simulink model "VFlexP_small"  (R2026a)
settings: Solver=ode23tb  StopTime=2  FixedStep=5e-5
model workspace (MAT data in the model file):
  DCop_DCBUCK : object (value not decoded)
  Grid_CCVSC_idx = [2; 3; 4; 5; 6; 7; 8; 9; 10; 11; 12]
  Grid_CCVSCs = 1
  Grid_CCVSCs_buses = 1
  Grid_CCVSCs_toM = [0 1 0 0 0 0 0 0 0 0 0 0 ... (781 elements, 71x11)]
  Grid_C_Lines = 0
  Grid_Cbuses = [0.00666666666667 0.00666666666667]
  Grid_DC : object (value not decoded)
  Grid_DCop_DCBUCK : object (value not decoded)
  Grid_DCop_DC_PES : object (value not decoded)
  Grid_DFIGs = 1
  Grid_DFIGs_buses = 1
  Grid_DGs : string (value not decoded)
  Grid_From_buses = 1
  Grid_GFls = 1
  Grid_GFls_buses = 1
  Grid_GFr_idx = 1
  Grid_GFrs = 1
  Grid_GFrs_buses = 1
  Grid_GFrs_toM = [1; 0]
  Grid_IG_idx = 1
  Grid_IGs = 1
  Grid_IGs_buses = 1
  Grid_IGs_toM = [1; 0; 0]
  Grid_L_Lines = 0.05
  Grid_L_Loads = [0 0]
  Grid_Lines_fromM : object (value not decoded)
  Grid_Lines_toM : object (value not decoded)
  Grid_Load_buses = [1; 2]
  Grid_Load_busesDC = []
  Grid_MSGs = 1
  Grid_MSGs_buses = 1
  Grid_Nbuses = 2
  Grid_PQ_gen = 3
  Grid_Ploads = [0.0075 0.0075]
  Grid_PloadsDC = []
  Grid_Ps_lf = 0.51232912
  Grid_Qloads = [0 0]
  Grid_Qs_lf = -0.00723209333333
  Grid_R_Lines = 0.005
  Grid_R_Loads = [2 2]
  Grid_R_Loads_DC = 0
  Grid_Rcf = [150 150]
  Grid_SCs = 1
  Grid_SCs_buses = 1
  Grid_SG_idx = 1
  Grid_SGs = 1
  Grid_SGs_buses = 1
  Grid_SGs_toM = [1; 0]
  Grid_To_buses = 2
  Grid_VCVSC_idx = [1; 2; 3; 4; 5; 6; 7; 8; 9; 10; 11; 12]
  Grid_VCVSCs = 1
  Grid_VCVSCs_buses = [1; 2; 3; 6; 8; 9; 12; 58; 59; 60; 63; 65]
  Grid_VCVSCs_toM = [1 0 0 0 0 0 0 0 0 0 0 0 ... (852 elements, 71x12)]
  Grid_VSM_idx = 2
  Grid_VSMs = 1
  Grid_VSMs_buses = 1
  Grid_VSMs_toM = [0; 1]
  Grid_admitt_matrix = [2.15353135314-19.7953135314i  -1.9801980198+19.801980198i; -1.9801980198+19.801980198i  2.15353135314-19.7953135314i]
  Grid_admitt_matrix_noloads = [1.98686468647-19.7953135314i  -1.9801980198+19.801980198i; -1.9801980198+19.801980198i  1.98686468647-19.7953135314i]
  Grid_bus = [1; 2]
  Grid_busDC_complexity = 1
  Grid_busDC_complexity_PF = 2
  Grid_bus_complexity = [1 1]
  Grid_bus_complexity_PF = [1 1]
  Grid_buses_lf = 1
  Grid_conductance_matrix = 0.00666666666667
  Grid_conductance_matrix_noloads = 0.00666666666667
  Grid_fref : object (value not decoded)
  Grid_gen_static_params : mBase (value not decoded)
  Grid_iPs_lf = 1.95187031336
  Grid_iQs_lf = -138.272551792
  Grid_iadmitt_matrix = [2.88165849328-0.0982918688642i  2.87905051706-0.123273862303i; 2.87905051706-0.123273862303i  2.88165849328-0.0982918688642i]
  Grid_iadmitt_matrix_noloads = [37.5012524798-37.4874983544i  37.4987475202-37.5125016456i; 37.4987475202-37.5125016456i  37.5012524798-37.4874983544i]
  Grid_iconductance_matrix = 150
  Grid_iconductance_matrix_noloads = 150
  Grid_init_OK_bool = 1
  Grid_intconv_PF : object (value not decoded)
  Grid_lf_op : op_report (value not decoded)
  Grid_lineDC_complexity = []
  Grid_lineDC_complexity_PF = []
  Grid_line_complexity = 1
  Grid_line_complexity_PF = 3
  Grid_loadDC_complexity = []
  Grid_loadDC_complexity_PF = []
  Grid_load_complexity = [3 3]
  Grid_load_complexity_PF = [4 4]
  Grid_opDC_CCVSC : object (value not decoded)
  Grid_opDC_VSM : object (value not decoded)
  Grid_opGFr : object (value not decoded)
  Grid_opVCVSC : object (value not decoded)
  Grid_op_CCVSC : object (value not decoded)
  Grid_op_IG : object (value not decoded)
  Grid_op_SG : object (value not decoded)
  Grid_op_VSM : object (value not decoded)
  Grid_shift_lines = 0
  Grid_tap_lines = 1
  Grid_v_buses_mod = [1 1]
  LinsysParamChangeStruct : Param1 (value not decoded)
  Lline = 0.01
  Rline = 1e-05
  linsys : object (value not decoded)
values from neighbouring files (symbols this model uses):
  block_idx = evalin(mdlWks, [bvarname Generators{i} '_idx'])    [fun_init_units_callback.m]
  Fb = areas    [fun_MATPOWER_to_Excel.m]
  Fi = evalin('base', get_param(block, 'Fi'))    [fun_init_GFr.m]    (also in fun_init_intconv_DC_VSM.m)
  Lf = evalin('base', get_param(block, 'Lf'))    [fun_init_GFr.m]    (also in fun_init_intconv_DC_VSM.m)
  Rf = evalin('base', get_param(block, 'Rf'))    [fun_init_GFr.m]    (also in fun_init_intconv_DC_VSM.m)
symbols that are objects in the model workspace (value not decoded): Grid_DCop_DC_PES, Grid_DCop_DCBUCK, Grid_op_CCVSC, Grid_op_IG, Grid_op_SG, Grid_op_VSM, Grid_opDC_CCVSC, Grid_opDC_VSM, Grid_opGFr, Grid_opVCVSC
undefined symbols (not defined in the file or in its folder): block_buses_DC, CCVSC_idx, Cf, costs, costs2, DFIGs_nodes, DiscIntNeverNeededParam, entity, From_nodes, grid_linsys, Grid_op_DFIG, Grid_op_DFIG_PQ, Grid_op_MSG, Grid_op_SC, Grid_op_VCVSC, Hv, initial_states_grid, Kic, Kiv, Kp_theta, Kp_w, Kpc, Kpv, last_send, Lc, m, Matrix_flux_to_i, mD, mp, MSGs_buses, Nbuses_DC, nq, op_VCVSC, Psche, Rc, rkq1, rkq2, SCs_buses, SCs_nodes, sec_control_structure, set_asked, set_DG_up, set_extra_satur, set_sending_cost, SGs_buses, SGs_nodes, Tf, To_nodes, VI_L, VI_R, WOF_Tf, xkq1, xkq2
libraries: simulink x1045, eeGeneralControl x12, eeTransforms x1, sl_discontinuities x1
(part 5 of 50)

== system VFlexP_small/Grid/Dynamic/Generators/DFIG ==
  note: do not rename this block, conditions to initialise the generator from PF result are set on this block's output
  note: port number 1
  note: port number 2
  elec_in : Inport
  v : Inport  Port=2
  AVR_Vmeas_Filter : Subsystem  mask{T_r=1e-6}
      mask prompts: T_r "Filter time constant"
      mask Display:
      | try
      |     dpoly(1, [T_r, 1])
      | catch
      | end
  AVR_Vmeas_Filter1 : Subsystem  mask{T_r=1e-6}
      mask prompts: T_r "Filter time constant"
      mask Display:
      | try
      |     dpoly(1, [T_r, 1])
      | catch
      | end
  AVR_Vmeas_Filter2 : Subsystem  mask{T_r=1e-6}
      mask prompts: T_r "Filter time constant"
      mask Display:
      | try
      |     dpoly(1, [T_r, 1])
      | catch
      | end
  Abs : Abs  SaturateOnIntegerOverflow=off
  Assignment : Assignment  NumberOfDimensions=2  DiagnosticForDimensions=Warning  IndexOptions=Assign all,Index vector (dialog)  Indices=1,block_idx  OutputSizes=1,1
  Atan2 : Trigonometry  SCDEnableBlockLinearizationSpecification=on  Operator=atan
  Cast To Boolean : DataTypeConversion  OutDataTypeStr=boolean  SaturateOnIntegerOverflow=off  RndMeth=Floor
  Cast To Double : DataTypeConversion  OutDataTypeStr=double  SaturateOnIntegerOverflow=off  RndMeth=Floor
  Cast To Double1 : DataTypeConversion  OutDataTypeStr=double  SaturateOnIntegerOverflow=off  RndMeth=Floor
  Complex to Magnitude-Angle1 : ComplexToMagnitudeAngle  Output=Magnitude
  Constant : Constant
  Constant10 : Constant  Commented=on  Value=1.83
  Constant2 : Constant  Value=zeros(1, length(block_buses))  VectorParams1D=off
  Constant6 : Constant  Commented=on  Value=-0.2
  Constant9 : Constant  Value=-0.89
  D : Constant  Commented=on  Value=11
  Decoupling vrdqFs : Subsystem
  Display{,1..11} (12 alike) : Display
  Divide1 : Product  Inputs=*/
  Divide2 : Product  Commented=on  Inputs=*/
  Divide4 : Product  Commented=on  Inputs=*/
  For Each Subsystem : Subsystem  TreatAsAtomicUnit=on
  From54 : From  Commented=on  GotoTag=v_to_follow_own
  From55 : From  Commented=on  GotoTag=omega_r
  From61 : From  Commented=on  GotoTag=s
  GSC Control : Subsystem
  Gain1 : Gain  Gain=-1
  Gain2 : Gain  Gain=1./Lm_pu
  Gain3 : Gain  Gain=Ps_lf(block_idx)
  Gain4 : Gain  Gain=-1
  Gain5 : Gain
  Gain6 : Gain  Commented=on  Gain=2
  Gain7 : Gain  Gain=-1
  Gain9 : Gain  Gain=1./Ps_lf(block_idx)
  Goto6 : Goto  Commented=on  GotoTag=omega_r_ref
  Integrator2 : Integrator  Commented=on  InitialCondition=Grid_op_DFIG.op.States(7).x'
  Integrator3 : Integrator  InitialCondition=Grid_op_DFIG.op.States(6).x'
  Integrator4 : Integrator  InitialCondition=Grid_op_DFIG.op.States(7).x'
  Manual Switch : ManualSwitch
  Matrix Concatenate : Concatenate  NumInputs=6  Mode=Multidimensional array
  Matrix Concatenate1 : Concatenate  NumInputs=3  Mode=Multidimensional array
  Memory : Memory  InitialCondition=1
  PI Q : Subsystem
  PI TE : Subsystem
  PI v : Subsystem  Commented=on
  PLL : Subsystem
  Product{,1..17} (18 alike) : Product
  RSC Control : Subsystem
  Rblade : Constant  Commented=on  Value=28
  Real-Imag to Complex : RealImagToComplex
  Real-Imag to Complex3 : RealImagToComplex
  Reference frame transform2 : Subsystem
  Reference frame transform3 : Subsystem
  Reference frame transform4 : Subsystem
  Reference frame transform5 : Subsystem
  Rotor Mechanical : Subsystem
  Scope4 : Scope
      settings: ActiveDisplayYMinimum=0.94445  ActiveDisplayYMaximum=0.94472  DataLoggingVariableName=ScopeData2
  Selector : Selector  NumberOfDimensions=2  InputPortWidth=3  IndexOptions=Index vector (dialog),Index vector (dialog)  Indices=1,block_idx  OutputSizes=1,1
  Selector1 : Selector  NumberOfDimensions=2  InputPortWidth=9  IndexOptions=Index vector (dialog),Select all  Indices=2,1  OutputSizes=1,1
  Selector2 : Selector  NumberOfDimensions=2  InputPortWidth=9  IndexOptions=Index vector (dialog),Select all  Indices=1,1  OutputSizes=1,1
  Selector3 : Selector  NumberOfDimensions=2  InputPortWidth=3  IndexOptions=Index vector (dialog),Index vector (dialog)  Indices=2,block_idx  OutputSizes=1,1
  Selector4 : Selector  NumberOfDimensions=2  InputPortWidth=3  IndexOptions=Index vector (dialog),Index vector (dialog)  Indices=3,block_idx  OutputSizes=1,1
  Selector5 : Selector  NumberOfDimensions=2  InputPortWidth=3  IndexOptions=Index vector (dialog),Index vector (dialog)  Indices=4,block_idx  OutputSizes=1,1
  Selector6 : Selector  NumberOfDimensions=2  InputPortWidth=3  IndexOptions=Index vector (dialog),Index vector (dialog)  Indices=5,block_idx  OutputSizes=1,1
  Selector7 : Selector  NumberOfDimensions=2  InputPortWidth=3  IndexOptions=Index vector (dialog),Index vector (dialog)  Indices=1,block_buses  OutputSizes=1,1
  Selector8 : Selector  NumberOfDimensions=2  InputPortWidth=3  IndexOptions=Index vector (dialog),Index vector (dialog)  Indices=2,block_buses  OutputSizes=1,1
  Signal Specification : SignalSpecification  Dimensions=[6 length(buses_lf)]
  Signal Specification1 : SignalSpecification  Dimensions=[3 length(block_buses)]
  Slip : Subsystem  Commented=on
      settings: PortSchema="{\"entries\":[{\"content\":{\"sides\":[{\"content\":{\"connectorIds\":[\"In1\",\"In2\"]},\"type\":\"ConnectorPlacement.EquallySpacedRectSide\",\"uuid\":\"76dc537b-974c-49aa-a996-6680dce67c21\"},{\"content\":{\"connectorIds\":[\"Out1\",\"Out2\"],\"side\":\"RIGHT\"},\"type\":\"ConnectorPlacement.EquallySpacedRectSide\",\"uuid\":\"b6b8ef66-c2c7-4653-a511-fa1c360be79f\"},{\"content\":{\"connectorIds\":[],\"side\":\"TOP\"},\"type\":\"ConnectorPlacement.EquallySpacedRectSide\",\"uuid\":\"e58a1e6b-6a60-4748-900e-908d64e83c02\"},{\"content\":{\"connectorIds\":[\"In3\"],\"side\":\"BOTTOM\"},\"type\":\"ConnectorPlacement.EquallySpacedRectSide\",\"uuid\":\"479d910e-b2a0-4bf0-91fd-3472aae41677\"}]},\"type\":\"ConnectorPlacement.EquallySpacedConnector\",\"uuid\":\"d6647aa7-5f1b-4486-ad87-47217a09b45e\"}],\"packageUris\":[\"http://schema.mathworks.com/mf0/Connector/R2020b\"],\"version\":\"1.0\"}"
  Stator circuit : Subsystem
  Subsystem : Subsystem
  Subsystem1 : Subsystem
  Sum : Sum  Inputs=-|-|-
  Sum{1,5..6,10..11,13} (6 alike) : Sum  Inputs=|-+
  Sum{4,9,12,14} (4 alike) : Sum  Inputs=|++
  Sum2 : Sum  Inputs=-|-|-
  Sum3 : Sum  Commented=on  Inputs=|+-
  Sum7 : Sum  Inputs=|+-
  TF_DELAY : Subsystem  Commented=on  mask{T_s=0.0001}
      mask prompts: T_s "Filter time constant"
      mask Display:
      | try
      |     dpoly(1, [T_s, 1])
      | catch
      | end
  TF_DELAY1 : Subsystem  mask{T_s=20E-3}
      mask prompts: T_s "Filter time constant"
      mask Display:
      | try
      |     dpoly(1, [T_s, 1])
      | catch
      | end
  Terminator{,1,3..8} (8 alike) : Terminator
  Vc control : Subsystem
  Vwind1 : Constant  Commented=on  Value=6
  Zero1 : Constant  Value=zeros(6, length(buses_lf))  VectorParams1D=off  OutDataTypeStr=Inherit: Inherit via back propagation
  connect : Subsystem
  lambda_opt : Gain  Commented=on  Gain=8
  psi->i1 : Subsystem
  tm : Integrator  InitialCondition=Grid_op_DFIG.op.States(24).x'  LimitOutput=on  UpperSaturationLimit=0  LowerSaturationLimit=-1
  trim_output : Subsystem
  w_ref_TF : Subsystem  Commented=on  mask{T_s=0.05}
      mask prompts: T_s "Filter time constant"
      mask Display:
      | try
      |     dpoly(1, [T_s, 1])
      | catch
      | end
  elec_out : Outport
  i : Outport  Port=2
  wires:
  From61/1 -> Slip/2(s)
  TF_DELAY/1(out) -> Gain6/1
  From55/1 -> TF_DELAY/1(in)
  D/1 -> Divide4/2
  Subsystem1/1(te) -> [te], Display10/1
  Divide4/1 -> w_ref_TF/1(in)
  w_ref_TF/1(out) -> Goto6/1
  Rblade/1 -> Divide2/2
  lambda_opt/1 -> Divide2/1
  Vwind1/1 -> Divide4/1, lambda_opt/1
  Sum7/1 -> PI Q/1(in)
  Sum4/1 -> AVR_Vmeas_Filter1/1(in)  "v"
  Sum5/1 -> AVR_Vmeas_Filter2/1(in)  "v"
  Real-Imag to Complex3/1 -> Complex to Magnitude-Angle1/1
  [v_q_PCC] -> Real-Imag to Complex3/2
  Complex to Magnitude-Angle1/1 -> AVR_Vmeas_Filter/1(in)  "v"
  [v_d_PCC] -> Real-Imag to Complex3/1
  Product5/1 -> Sum5/1
  [v_d_PCC] -> Product1/1, Product5/1  "vod"
  Product3/1 -> Sum4/2
  [id_out] -> Product1/2, Product6/2  "iod"
  [v_q_PCC] -> Product6/1, Product3/1  "voq"
  Product6/1 -> Sum5/2
  Product1/1 -> Sum4/1
  [iq_out] -> Product3/2, Product5/2  "ioq"
  tm/1 -> Manual Switch/1
  Signal Specification/1 -> elec_out/1
  Gain4/1 -> Reference frame transform3/2(theta)
  [vaq] -> Stator circuit/6(vaq)
  Constant9/1 -> Manual Switch/2
  Sum/1 -> Reference frame transform5/1(in_d)
  Sum2/1 -> Reference frame transform5/3(in_q)
  PLL/1(theta_rad_pll) -> [theta], Terminator1/1
  For Each Subsystem/1(Out1) -> i/1
  Reference frame transform5/1(out_d) -> connect/1(id), [id_out]
  Product/1 -> Sum1/1
  [v_d_PCC] -> Stator circuit/1(vsd)
  trim_output/2(Out2) -> Terminator6/1
  ? -> Sum2/3
  [vrd_] -> Decoupling vrdqFs/2(Vrd')
  [vad] -> Stator circuit/5(vad)
  Selector5/1 -> [Q_s_to_follow_own]
  [iad] -> GSC Control/4(iad)
  Vc control/1(iad_ref) -> [iad_ref]
  psi->i1/5(irq) -> [irq], Subsystem1/3(irq)
  Real-Imag to Complex/1 -> Abs/1
  [vrd] -> Vc control/2(vrd)
  [vad] -> Vc control/6(vad)
  [te] -> Rotor Mechanical/1(te)
  [omega_ref] -> Terminator/1  "ref_omega"
  [vrd] -> Stator circuit/3(vrd)
  Assignment/1 -> Signal Specification/1
  Reference frame transform2/2(vrq) -> [vrq]
  [v_q_PCC] -> PLL/1(vdq0_meas)
  Decoupling vrdqFs/1(vrd_Fs) -> Reference frame transform2/1(vrd_Fs)
  GSC Control/1(vad) -> [vad]
  [v_q_PCC] -> Stator circuit/2(vsq)
  psi->i1/6(iad) -> [iad]
  [iaq] -> Vc control/9(iaq)
  Selector2/1 -> Divide1/2, Real-Imag to Complex/1
  GSC Control/2(vaq) -> [vaq]
  [vsq] -> GSC Control/2(vsq)
  RSC Control/2(vrq') -> [vrq_]
  RSC Control/1(vrd') -> [vrd_]
  [phi] -> Gain1/1
  [vrq] -> Vc control/3(vrq)
  Divide1/1 -> Atan2/1
  [ws] -> Decoupling vrdqFs/4(ws)
  Reference frame transform2/1(vrd) -> [vrd]
  PLL/2(omega_pu_pll) -> Terminator3/1
  [vrq_] -> Decoupling vrdqFs/6(vrq')
  psi->i1/3(isq) -> [isq]
  [iad_ref] -> GSC Control/3(iad_ref)
  ? -> Sum/3
  PLL/3(Freq_Hz_pll) -> Terminator4/1
  Constant/1 -> Vc control/1(Vc_2_ref)
  [iad] -> Vc control/8(iad)
  Gain2/1 -> Decoupling vrdqFs/5(ism)
  [vdout] -> Reference frame transform3/1(in_d)
  [theta] -> Gain4/1
  Gain9/1 -> Matrix Concatenate/2
  Reference frame transform3/2(out_q) -> [vsq], [v_q_PCC]
  [P_s] -> Gain9/1  "P_s"
  [isd] -> Sum/1
  psi->i1/4(ird) -> [ird], Subsystem1/2(ird)
  Matrix Concatenate1/1 -> Signal Specification1/1
  trim_output/4(Out4) -> Terminator8/1
  Selector8/1 -> [vqout], trim_output/4(vq)
  Constant2/1 -> Matrix Concatenate1/3
  [irq] -> Reference frame transform4/3(irq)
  [vqout] -> Reference frame transform3/3(in_q)
  trim_output/3(Out3) -> Terminator7/1
  Cast To Boolean/1 -> [connect]
  [ws] -> Stator circuit/8(ws)
  v/1 -> Selector8/1, Selector7/1
  Rotor Mechanical/1(s) -> Product/1, [s]
  [i] -> Stator circuit/7(i)
  Signal Specification1/1 -> For Each Subsystem/1(In1)
  [vsd] -> GSC Control/1(vsd)
  Reference frame transform4/2(out_q) -> RSC Control/4(irq_Fs_meas), Decoupling vrdqFs/1(irq_Fs)
  Atan2/1 -> [phi], Display2/1
  [ws] -> GSC Control/7(ws)
  Selector7/1 -> trim_output/3(vd), [vdout]
  Gain5/1 -> Reference frame transform5/2(theta)
  elec_in/1 -> Selector6/1, Selector5/1, Selector4/1, Selector3/1, Selector/1
  connect/2(iq_real) -> trim_output/2(iq), Matrix Concatenate1/2
  [connect] -> Cast To Double1/1
  Cast To Double/1 -> Matrix Concatenate/6
  Cast To Double1/1 -> Matrix Concatenate/5
  [phi] -> Reference frame transform2/2(phi)
  Selector6/1 -> Cast To Boolean/1
  [Q_s] -> Matrix Concatenate/4  "Q_s"
  connect/1(id_real) -> trim_output/1(id), Matrix Concatenate1/1
  [ird] -> Reference frame transform4/1(ird)
  psi->i1/7(iaq) -> [iaq]
  [vrq] -> Stator circuit/4(vrq)
  psi->i1/1(i) -> Display1/1, [i]
  trim_output/1(Out1) -> Terminator5/1
  [ws] -> Matrix Concatenate/1  "omega"
  Zero1/1 -> Assignment/1
  Selector/1 -> [omega_to_follow_own]
  Selector3/1 -> Gain3/1
  Selector4/1 -> [v_to_follow_own]
  Gain3/1 -> [P_s_to_follow_own]
  [vaq] -> Vc control/7(vaq)
  [ird] -> Vc control/4(ird)
  Matrix Concatenate/1 -> Assignment/2
  [iaq] -> GSC Control/6(iaq)
  [isq] -> Sum2/1
  [omega_ref] -> Rotor Mechanical/3(ws), Product/2, [ws], Sum1/2
  Reference frame transform5/2(out_q) -> connect/2(iq), [iq_out]
  [theta] -> Gain5/1
  psi->i1/2(isd) -> [isd]
  Stator circuit/1(psi) -> Display/1, psi->i1/1(psi), Subsystem1/1(psisdq), Selector1/1, Selector2/1
  [connect] -> connect/3(connect)
  [s] -> Stator circuit/9(s)
  Decoupling vrdqFs/2(vrq_Fs) -> Reference frame transform2/3(vrq_Fs)
  Reference frame transform3/1(out_d) -> [vsd], [v_d_PCC]
  [s] -> Decoupling vrdqFs/3(s)
  [iad] -> Sum/2
  AVR_Vmeas_Filter/1(out) -> [Vt_mod], Matrix Concatenate/3  "v"
  Selector1/1 -> Divide1/1, Real-Imag to Complex/2
  [connected] -> Memory/1
  [irq] -> Vc control/5(irq)
  connect/3(connected) -> [connected]
  [iaq] -> Sum2/2
  Gain1/1 -> Reference frame transform4/2(phi)
  Memory/1 -> Cast To Double/1
  [isd] -> Product4/2, Product9/2  "iod"
  [isq] -> Product7/2, Product8/2  "ioq"
  Product9/1 -> Sum10/2
  Product7/1 -> Sum9/2
  [v_d_PCC] -> Product4/1, Product8/1  "vod"
  Sum10/1 -> [Q_stator], Display7/1  "v"
  [v_q_PCC] -> Product9/1, Product7/1  "voq"
  Product4/1 -> Sum9/1
  Sum9/1 -> Display8/1, [P_stator]  "v"
  Product8/1 -> Sum10/1
  Product12/1 -> Sum11/1
  Sum12/1 -> [P_rotor], Display6/1  "v"
  Product10/1 -> Sum12/1
  [vrq] -> Product11/1, Product13/1  "voq"
  Sum11/1 -> Display5/1, [Q_rotor]  "v"
  [vrd] -> Product12/1, Product10/1  "vod"
  Product11/1 -> Sum12/2
  Product13/1 -> Sum11/2
  [irq] -> Product12/2, Product11/2  "ioq"
  [ird] -> Product13/2, Product10/2  "iod"
  [iad] -> Product14/2, Product17/2  "iod"
  [iaq] -> Product15/2, Product16/2  "ioq"
  Product17/1 -> Sum13/2
  Product15/1 -> Sum14/2
  [vad] -> Product14/1, Product16/1  "vod"
  Sum13/1 -> [Q_gsc], Display3/1  "v"
  [vaq] -> Product17/1, Product15/1  "voq"
  Product14/1 -> Sum14/1
  Sum14/1 -> Display4/1, [P_gsc]  "v"
  Product16/1 -> Sum13/1
  Constant6/1 -> Slip/1(s_ref)
  Slip/2(Te) -> ?
  Integrator3/1 -> Sum7/2
  AVR_Vmeas_Filter1/1(out) -> [P_s], Display9/1  "v"
  AVR_Vmeas_Filter2/1(out) -> [Q_s]  "v"
  Subsystem/1(Out1) -> Gain7/1
  Product2/1 -> Subsystem/1(omega_r)
  [omega_r] -> TF_DELAY1/1(in)
  Sum3/1 -> PI v/1(in)
  From54/1 -> Sum3/1
  Sum1/1 -> [omega_r], Scope4/1
  Abs/1 -> Gain2/1
  Integrator2/1 -> Sum3/2
  Gain7/1 -> Display11/1, [Te_ref]
  [Te_ref] -> Sum6/1
  [te] -> Sum6/2
  Sum6/1 -> PI TE/1(in)
  TF_DELAY1/1(out) -> Product2/2, Product2/1
  [Q_s_to_follow_own] -> Sum7/1
  Integrator4/1 -> GSC Control/5(iaq_ref)
  PI TE/1(out) -> RSC Control/3(irq_Fs_ref)
  Reference frame transform4/1(out_d) -> RSC Control/2(ird_Fs_meas), Decoupling vrdqFs/7(ird_Fs)
  PI Q/1(out) -> RSC Control/1(ird_Fs_ref)
  Manual Switch/1 -> Rotor Mechanical/2(tm)

== system VFlexP_small/Grid/Dynamic/Generators/GFl ==
  note: do not rename this block, conditions to initialise the generator from PF result are set on this block's output
  note: port number 1
  note: port number 2
  elec_in : Inport
  v : Inport  Port=2
  Assignment : Assignment  NumberOfDimensions=2  DiagnosticForDimensions=Warning  IndexOptions=Assign all,Index vector (dialog)  Indices=1,block_idx  OutputSizes=1,1
  CC : Subsystem  Variant=on  VariantControlMode=label  LabelModeActiveChoice=static
  Cast To Boolean1 : DataTypeConversion  OutDataTypeStr=boolean  SaturateOnIntegerOverflow=off  RndMeth=Floor
  Cast To Double : DataTypeConversion  OutDataTypeStr=double  SaturateOnIntegerOverflow=off  RndMeth=Floor
  Cast To Double1 : DataTypeConversion  OutDataTypeStr=double  SaturateOnIntegerOverflow=off  RndMeth=Floor
  Cast To Double2 : DataTypeConversion  OutDataTypeStr=double  SaturateOnIntegerOverflow=off  RndMeth=Floor
  Complex to Magnitude-Angle : ComplexToMagnitudeAngle  Output=Angle
  Complex to Magnitude-Angle1 : ComplexToMagnitudeAngle  Output=Magnitude
  Constant : Constant  Value=zeros(1, length(block_buses))  VectorParams1D=off
  For Each Subsystem : Subsystem  TreatAsAtomicUnit=on
  Gain : Gain  Gain=-1
  Gain3 : Gain  Commented=through  Gain=iQs_lf(CCVSC_idx)
  Gain4 : Gain  Commented=through  Gain=iPs_lf(CCVSC_idx)
  LPF : Subsystem
  LPF1 : Subsystem
  LPF2 : Subsystem
  LPF3 : Subsystem
  LPF_d : Subsystem  Commented=through
  LPF_q : Subsystem  Commented=through
  Matrix Concatenate : Concatenate  NumInputs=6  Mode=Multidimensional array
  Matrix Concatenate1 : Concatenate  NumInputs=3  Mode=Multidimensional array
  Memory : Memory  InitialCondition=1
  Memory1 : Memory  InitialCondition=1
  Memory2 : Memory  InitialCondition=1
  PC : Subsystem
      settings: PortSchema="{\"entries\":[{\"content\":{\"sides\":[{\"content\":{\"connectorIds\":[\"In1\",\"In2\",\"In3\",\"In4\"]},\"type\":\"ConnectorPlacement.EquallySpacedRectSide\",\"uuid\":\"7748ce6f-2dcc-431c-b3ea-0be9c3088b1d\"},{\"content\":{\"connectorIds\":[\"In5\",\"Out1\",\"Out2\"],\"side\":\"RIGHT\"},\"type\":\"ConnectorPlacement.EquallySpacedRectSide\",\"uuid\":\"af86fd8d-043b-4d20-8ee8-e7a977d706a8\"},{\"content\":{\"connectorIds\":[],\"side\":\"TOP\"},\"type\":\"ConnectorPlacement.EquallySpacedRectSide\",\"uuid\":\"807e0dc6-0d59-4ea5-9557-3ccfd29c2ad0\"}]},\"type\":\"ConnectorPlacement.EquallySpacedConnector\",\"uuid\":\"c7fe00c5-0a0a-4038-b7ac-e659fb2aa4a7\"}],\"packageUris\":[\"http://schema.mathworks.com/mf0/Connector/R2020b\"],\"version\":\"1.0\"}"
  PLL : Subsystem  Variant=on  VariantControlMode=label  LabelModeActiveChoice=dynamic
  Product{,1..3} (4 alike) : Product
  Real-Imag to Complex : RealImagToComplex
  Real-Imag to Complex1 : RealImagToComplex
  Reference frame transform3 : Subsystem
  Reference_frame_transform1 : Subsystem
  Selector : Selector  NumberOfDimensions=2  InputPortWidth=3  IndexOptions=Index vector (dialog),Index vector (dialog)  Indices=1,block_idx  OutputSizes=1,1
  Selector1 : Selector  NumberOfDimensions=2  InputPortWidth=3  IndexOptions=Index vector (dialog),Index vector (dialog)  Indices=2,block_idx  OutputSizes=1,1
  Selector2 : Selector  NumberOfDimensions=2  InputPortWidth=3  IndexOptions=Index vector (dialog),Index vector (dialog)  Indices=3,block_idx  OutputSizes=1,1
  Selector3 : Selector  NumberOfDimensions=2  InputPortWidth=3  IndexOptions=Index vector (dialog),Index vector (dialog)  Indices=4,block_idx  OutputSizes=1,1
  Selector4 : Selector  NumberOfDimensions=2  InputPortWidth=3  IndexOptions=Index vector (dialog),Index vector (dialog)  Indices=5,block_idx  OutputSizes=1,1
  Selector5 : Selector  NumberOfDimensions=2  InputPortWidth=3  IndexOptions=Index vector (dialog),Index vector (dialog)  Indices=1,block_buses  OutputSizes=1,1
  Selector6 : Selector  NumberOfDimensions=2  InputPortWidth=3  IndexOptions=Index vector (dialog),Index vector (dialog)  Indices=2,block_buses  OutputSizes=1,1
  Selector7 : Selector  InputPortWidth=length(fref.ref_units)  IndexOptions=Index vector (dialog)  Indices=block_fref  OutputSizes=1
  Signal Specification : SignalSpecification  Dimensions=[6 length(buses_lf)]
  Signal Specification1 : SignalSpecification  Dimensions=[3 length(block_buses)]
  Sum : Sum  Inputs=|++
  Sum1 : Sum  Inputs=|-+
  Terminator{,3..5} (4 alike) : Terminator
  Zero1 : Constant  Value=zeros(6, length(buses_lf))  VectorParams1D=off  OutDataTypeStr=Inherit: Inherit via back propagation
  connect : Subsystem
  trim_output : Subsystem
  elec_out : Outport
  i : Outport  Port=2
  wires:
  LPF_q/1(Out1) -> Gain3/1
  LPF_d/1(Out1) -> Gain4/1
  [voutangle] -> PLL/1(voutangle)
  [Q_s_to_follow_own] -> PC/4(vodi2)
  [P_s_to_follow_own] -> PC/3(vodi1)
  connect/3(connected) -> Cast To Double/1
  CC/2(iqiref) -> Reference_frame_transform1/2(qin)  "ioq"
  CC/1(idiref) -> Reference_frame_transform1/1(din)  "iod"
  Reference frame transform3/2(out_q) -> [voq]
  PLL/1(theta) -> [theta]
  [omega_ref] -> Selector7/1
  [voq] -> PLL/2(vq)
  [theta] -> Reference_frame_transform1/3(theta)
  Gain/1 -> Reference frame transform3/2(theta)
  [theta] -> Gain/1
  PC/2(Output1) -> CC/2(iqref)  "ioq"
  PC/1(Output) -> CC/1(idref)  "iod"
  [v_q_PCC] -> Product3/1  "voq"
  [v_d_PCC] -> Product2/1  "vod"
  [ioq] -> Product1/2  "ioq"
  [iod] -> Product/2  "iod"
  [v_d_PCC] -> Product/1  "vod"
  Gain3/1 -> [Q_s]
  Gain4/1 -> [P_s]
  Product/1 -> Sum/1
  Product3/1 -> Sum1/2
  Product1/1 -> Sum/2
  Product2/1 -> Sum1/1
  [ioq] -> Product2/2  "ioq"
  [iod] -> Product3/2  "iod"
  Sum1/1 -> LPF_q/1(In1)
  Sum/1 -> LPF_d/1(In1)
  [v_q_PCC] -> Product1/1  "voq"
  Reference frame transform3/1(out_d) -> [vod]  "v CCVSC"
  [voq] -> PC/2(voq), CC/4(voq)
  [vod] -> PC/1(vodi), CC/3(vod)
  Real-Imag to Complex/1 -> Complex to Magnitude-Angle/1
  Complex to Magnitude-Angle/1 -> [voutangle]
  PLL/2(omega_point) -> PC/5(omega), CC/5(omega), [omega]  "\\omega CCVSC"
  Reference_frame_transform1/2(qout) -> connect/2(iq)
  Reference_frame_transform1/1(dout) -> connect/1(id)
  [vqout] -> LPF3/1(In1)
  Selector3/1 -> [Q_s_to_follow_own]
  Selector2/1 -> [v_to_follow_own]
  Selector/1 -> [omega_to_follow_own]
  [omega] -> Matrix Concatenate/1  "omega"
  [P_s] -> Matrix Concatenate/2  "P_s"
  [Q_s] -> Matrix Concatenate/4  "Q_s"
  [connected] -> Memory/1
  [connect] -> Memory1/1
  Cast To Double/1 -> [connected]
  [connect] -> connect/3(connect)
  [vdout] -> LPF2/1(In1)
  connect/1(id_real) -> [iod], trim_output/1(id), Matrix Concatenate1/1
  connect/2(iq_real) -> [ioq], trim_output/2(iq), Matrix Concatenate1/2
  LPF3/1(Out1) -> [v_q_PCC]
  LPF2/1(Out1) -> [v_d_PCC]
  [v_d_PCC] -> Real-Imag to Complex1/1  "vod"
  [v_q_PCC] -> Real-Imag to Complex1/2  "voq"
  Real-Imag to Complex1/1 -> Complex to Magnitude-Angle1/1
  Complex to Magnitude-Angle1/1 -> Matrix Concatenate/3
  [v_d_PCC] -> LPF/1(In1)  "vod"
  [v_q_PCC] -> LPF1/1(In1)  "voq"
  Selector4/1 -> Cast To Boolean1/1
  Cast To Boolean1/1 -> Memory2/1
  Cast To Double1/1 -> Matrix Concatenate/5
  Cast To Double2/1 -> Matrix Concatenate/6
  Zero1/1 -> Assignment/1
  Signal Specification/1 -> elec_out/1
  Assignment/1 -> Signal Specification/1
  Matrix Concatenate/1 -> Assignment/2
  elec_in/1 -> Selector4/1, Selector3/1, Selector2/1, Selector1/1, Selector/1
  Matrix Concatenate1/1 -> Signal Specification1/1
  Signal Specification1/1 -> For Each Subsystem/1(In1)
  Constant/1 -> Matrix Concatenate1/3
  For Each Subsystem/1(Out1) -> i/1
  trim_output/1(Out1) -> Terminator/1
  trim_output/3(Out3) -> Terminator4/1
  trim_output/2(Out2) -> Terminator3/1
  trim_output/4(Out4) -> Terminator5/1
  Selector5/1 -> trim_output/3(vd), [vdout]
  Selector6/1 -> trim_output/4(vq), [vqout]
  v/1 -> Selector6/1, Selector5/1
  Memory/1 -> Cast To Double2/1
  Selector1/1 -> [P_s_to_follow_own]
  Memory1/1 -> Cast To Double1/1
  Memory2/1 -> [connect]
  LPF/1(Out1) -> Reference frame transform3/1(in_d), Real-Imag to Complex/1
  LPF1/1(Out1) -> Real-Imag to Complex/2, Reference frame transform3/3(in_q)
  Selector7/1 -> PLL/3(omega)

== system VFlexP_small/Grid/Dynamic/Generators/GFr ==
  note: port number 1
  note: do not rename this block, conditions to initialise the generator from PF result are set on this block's output
  note: port number 2
  elec_in : Inport
  v : Inport  Port=2
  AND : Logic  IconShape=distinctive  AllPortsSameDT=off  OutDataTypeStr=boolean
  AND1 : Logic  IconShape=distinctive  AllPortsSameDT=off  OutDataTypeStr=boolean
  AND2 : Logic  IconShape=distinctive  AllPortsSameDT=off  OutDataTypeStr=boolean
  Abs{,1..3} (4 alike) : Abs  ZeroCross=off  SaturateOnIntegerOverflow=off
  Assignment : Assignment  NumberOfDimensions=2  DiagnosticForDimensions=Warning  IndexOptions=Assign all,Index vector (dialog)  Indices=1,block_idx  OutputSizes=1,1
  Atan2 : Trigonometry  Operator=atan2
  Cast To Boolean : DataTypeConversion  OutDataTypeStr=boolean  SaturateOnIntegerOverflow=off  RndMeth=Floor
  Cast To Double : DataTypeConversion  OutDataTypeStr=double  SaturateOnIntegerOverflow=off  RndMeth=Floor
  Cast To Double1 : DataTypeConversion  OutDataTypeStr=double  SaturateOnIntegerOverflow=off  RndMeth=Floor
  Cast To Double2 : DataTypeConversion  OutDataTypeStr=double  SaturateOnIntegerOverflow=off  RndMeth=Floor
  Compare To Constant : simulink/Logic and Bit Operations/Compare To Constant  relop=<=  const=0.001  OutDataTypeStr=boolean  ZeroCross=off
  Compare To Constant1 : simulink/Logic and Bit Operations/Compare To Constant  relop=<=  const=0.01  OutDataTypeStr=boolean  ZeroCross=off
  Compare To Constant2 : simulink/Logic and Bit Operations/Compare To Constant  relop=<=  const=0.2  OutDataTypeStr=boolean  ZeroCross=off
  Compare To Constant3 : simulink/Logic and Bit Operations/Compare To Constant  relop=>  const=4  OutDataTypeStr=boolean  ZeroCross=off
  Complex to Magnitude-Angle1 : ComplexToMagnitudeAngle  Output=Magnitude
  Complex to Real-Imag : ComplexToRealImag
  Conjugate : Math  Operator=conj  SignedPower=on  RndMeth=Zero
  Constant : Constant  Value=zeros(1, length(block_buses))  VectorParams1D=off
  Constant1 : Constant  Value=Grid_opVCVSC.Pd
  For Each Subsystem : Subsystem  TreatAsAtomicUnit=on
  Gain : Gain  Gain=mD
  Gain1 : Gain  Gain=-1
  Gain2 : Gain  Gain=-1
  Integrator : Integrator  ExternalReset=falling  InitialCondition=Grid_opGFr.IntConnect
  LPF : Subsystem  Commented=through
  LPF1 : Subsystem  Commented=through
  LPF_P : Subsystem
  LPF_omega : Subsystem
  LPF_v : Subsystem
  Matrix Concatenate : Concatenate  NumInputs=6  Mode=Multidimensional array
  Matrix Concatenate1 : Concatenate  NumInputs=3  Mode=Multidimensional array
  Memory : Memory  InitialCondition=1
  Memory1 : Memory  InitialCondition=1
  Memory2 : Memory  InitialCondition=1
  NOT1 : Logic  Operator=NOT  IconShape=distinctive  AllPortsSameDT=off  OutDataTypeStr=boolean
  OR : Logic  Operator=OR  Inputs=3  IconShape=distinctive  AllPortsSameDT=off  OutDataTypeStr=boolean
  PC : Subsystem  mask(PC_VCVSC){Tf=Tf, mp=mp, nq=nq}
      mask prompts: Tf "Low-pass filter time constant (s)"; mp "Droop coefficient mp"; nq "Droop coefficient nq"
      mask help: Power controller of a grid-forming converter, including the droop control and low-pass filters for the power measurements.
      mask init: same as VFlexP_small/Grid/Dynamic/DCAC converters/DC_VCVSC/PC
  PI_synchro_f : Subsystem
  PI_synchro_v : Subsystem
  Product : Product
  Product1 : Product  OutDataTypeStr=double
  Product2 : Product  OutDataTypeStr=double
  Product3 : Product
  RL out : Subsystem  Variant=on  VariantControlMode=label  LabelModeActiveChoice=dynamic  mask{dynamic=Dynamic, R=R_out, L=L_out}
      mask prompts: dynamic "Dynamic behavior"; R "Series resistance (p.u.)"; L "Inductance (p.u.)"
      mask init:
      | invL = 1./L;
      | vssBlk = gcb;
      | switch dynamic
      |     case "Static"
      |         set_param(vssBlk, 'LabelModeActiveChoice', 'static');
      |     case "Dynamic"
      |         set_param(vssBlk, 'LabelModeActiveChoice', 'dynamic');
      |     case "Static omega"
      |         set_param(vssBlk, 'LabelModeActiveChoice', 'static_omega');
      | end
      mask TypeOptions dynamic: Static | Dynamic | Static omega
  Real-Imag to Complex : RealImagToComplex
  Real-Imag to Complex1 : RealImagToComplex
  Real-Imag to Complex3 : RealImagToComplex
  Reference frame transform1 : Subsystem
  Reference frame transform2 : Subsystem
  Reference frame transform3 : Subsystem
  Scope : Scope
      settings: ActiveDisplayYMinimum=0.9  ActiveDisplayYMaximum=1.1
  Selector : Selector  NumberOfDimensions=2  InputPortWidth=3  IndexOptions=Index vector (dialog),Index vector (dialog)  Indices=1,block_idx  OutputSizes=1,1
  Selector1 : Selector  NumberOfDimensions=2  InputPortWidth=3  IndexOptions=Index vector (dialog),Index vector (dialog)  Indices=2,block_idx  OutputSizes=1,1
  Selector2 : Selector  NumberOfDimensions=2  InputPortWidth=3  IndexOptions=Index vector (dialog),Index vector (dialog)  Indices=3,block_idx  OutputSizes=1,1
  Selector3 : Selector  NumberOfDimensions=2  InputPortWidth=3  IndexOptions=Index vector (dialog),Index vector (dialog)  Indices=4,block_idx  OutputSizes=1,1
  Selector4 : Selector  NumberOfDimensions=2  InputPortWidth=3  IndexOptions=Index vector (dialog),Index vector (dialog)  Indices=5,block_idx  OutputSizes=1,1
  Selector5 : Selector  NumberOfDimensions=2  InputPortWidth=3  IndexOptions=Index vector (dialog),Index vector (dialog)  Indices=1,block_buses  OutputSizes=1,1
  Selector6 : Selector  NumberOfDimensions=2  InputPortWidth=3  IndexOptions=Index vector (dialog),Index vector (dialog)  Indices=2,block_buses  OutputSizes=1,1
  Selector7 : Selector  InputPortWidth=length(fref.ref_units)  IndexOptions=Index vector (dialog)  Indices=block_fref  OutputSizes=1
  Selector8 : Selector  InputPortWidth=length(fref.ref_units)  IndexOptions=Index vector (dialog)  Indices=block_fref  OutputSizes=1
  Signal Specification : SignalSpecification  Dimensions=[6 length(buses_lf)]
  Signal Specification1 : SignalSpecification  Dimensions=[3 length(block_buses)]
  Sum : Sum  Inputs=|+-
  Sum1 : Sum  Inputs=|++
  Sum11 : Sum  Inputs=|++
  Sum12 : Sum  Inputs=|++
  Sum2 : Sum  Inputs=-+|
  Sum3 : Sum  Inputs=|+-
  Sum4 : Sum  Inputs=|+-
  Sum8 : Sum  Inputs=++|
  Switch2 : Switch  Criteria=u2 > Threshold  SaturateOnIntegerOverflow=off  InputSameDT=off
  Switch3 : Switch  Criteria=u2 > Threshold  SaturateOnIntegerOverflow=off  InputSameDT=off
  Terminator{,1..5} (6 alike) : Terminator
  VCC : Subsystem  Variant=on  VariantControlMode=label  LabelModeActiveChoice=static
  VI : Subsystem  mask{L=VI_L, R=VI_R, Tf=WOF_Tf}
      mask prompts: L "Inductance (pu)"; R "Resistance (pu)"; Tf "WOF time constant (s)"
      mask init: same as VFlexP_small/Grid/Dynamic/DCAC converters/DC_VCVSC/VI
  Zero : Constant  Value=0  OutDataTypeStr=Inherit: Inherit via back propagation
  Zero1 : Constant  Value=zeros(6, length(buses_lf))  VectorParams1D=off  OutDataTypeStr=Inherit: Inherit via back propagation
  connect : Subsystem
  frame : Integrator  InitialCondition=Grid_opGFr.frame  IgnoreLimit=on
  iV : Integrator  InitialCondition=Grid_opGFr.iV
  trim_output : Subsystem
  vod : Sum  Inputs=++|
  elec_out : Outport
  i : Outport  Port=2
  wires:
  Sum8/1 -> VCC/2(voqref)
  vod/1 -> VCC/1(vodref)
  [omega] -> VI/3(omega)
  [ioq] -> VI/2(iq)
  [iod] -> VI/1(id)
  Gain2/1 -> Reference frame transform2/2(theta)
  [theta] -> Gain2/1
  connect/3(connected) -> [connected]
  [omega] -> Sum2/2  "omega"
  [omega_ref] -> Selector7/1  "ref_omega"
  RL out/1(id) -> connect/1(id)
  [theta] -> Gain1/1
  Gain1/1 -> Reference frame transform1/2(theta)
  [ioq] -> VCC/4(ioq)
  [iod] -> VCC/3(iod)
  Zero/1 -> Sum8/2
  [vodref] -> vod/2
  [omega] -> VCC/5(omega)
  [theta] -> Reference frame transform3/2(theta)
  PC/1(Out1) -> [omega]
  PC/2(Out2) -> [vodref]
  [iod] -> PC/2(iodi)
  [ioq] -> PC/1(ioq)
  Reference frame transform1/2(out_q) -> [ioq]
  Reference frame transform3/1(out_d) -> RL out/1(v_in_d)
  Reference frame transform3/2(out_q) -> RL out/3(v_in_q)
  RL out/2(iq) -> connect/2(iq)
  Reference frame transform1/1(out_d) -> [iod]
  VI/1(vd) -> vod/1
  VI/2(vq) -> Sum8/1
  connect/1(id_real) -> trim_output/1(id), Matrix Concatenate1/1, Reference frame transform1/1(in_d)
  connect/2(iq_real) -> trim_output/2(iq), Matrix Concatenate1/2, Reference frame transform1/3(in_q)
  RL out/3(v_outd) -> Terminator1/1
  RL out/4(v_outq) -> Terminator2/1
  Selector3/1 -> [Q_s_to_follow]
  Selector/1 -> [omega_to_follow]
  Selector2/1 -> [v_to_follow]
  [Q_s] -> Matrix Concatenate/4
  [P_s] -> Matrix Concatenate/2  "P_s"
  Complex to Magnitude-Angle1/1 -> Matrix Concatenate/3  "v"
  Matrix Concatenate/1 -> Assignment/2
  elec_in/1 -> Selector4/1, Selector3/1, Selector2/1, Selector1/1, Selector/1
  Assignment/1 -> Signal Specification/1
  [connect] -> Cast To Double1/1
  [connected] -> Memory/1
  Selector4/1 -> Memory1/1
  Cast To Double/1 -> Matrix Concatenate/6
  Cast To Double1/1 -> Matrix Concatenate/5
  Reference frame transform2/1(out_d) -> LPF/1(In1)
  Reference frame transform2/2(out_q) -> LPF1/1(In1)
  [v_d_PCC] -> Real-Imag to Complex/1
  [v_q_PCC] -> Real-Imag to Complex/2
  [vod] -> Real-Imag to Complex1/1
  [voq] -> Real-Imag to Complex1/2
  Real-Imag to Complex1/1 -> Abs1/1, Conjugate/1
  Real-Imag to Complex/1 -> Abs/1, Product/1
  Conjugate/1 -> Product/2
  Product/1 -> Complex to Real-Imag/1
  Complex to Real-Imag/2 -> Atan2/1
  Complex to Real-Imag/1 -> Atan2/2
  Abs/1 -> Compare To Constant2/1, Sum3/1
  Sum3/1 -> Abs2/1, Product1/2
  Product1/1 -> PI_synchro_v/1(In1)
  Product2/1 -> PI_synchro_f/1(In1)
  Atan2/1 -> Abs3/1, Product2/2
  Cast To Boolean/1 -> [connect]
  Abs1/1 -> Sum3/2
  Signal Specification/1 -> elec_out/1
  Abs2/1 -> Compare To Constant/1
  Compare To Constant/1 -> AND/2
  Abs3/1 -> Compare To Constant1/1
  Compare To Constant1/1 -> AND/1
  AND/1 -> OR/1
  OR/1 -> Memory2/1
  [connected] -> OR/3
  Memory2/1 -> [safe_to_connect]
  [vqout] -> Reference frame transform2/3(in_q), RL out/4(v_out_q)
  LPF/1(Out1) -> [v_d_PCC]
  LPF1/1(Out1) -> [v_q_PCC]
  [vdout] -> RL out/2(v_out_d), Reference frame transform2/1(in_d)
  Matrix Concatenate1/1 -> Signal Specification1/1
  Constant/1 -> Matrix Concatenate1/3
  For Each Subsystem/1(Out1) -> i/1
  Signal Specification1/1 -> For Each Subsystem/1(In1)
  [v_d_PCC] -> PC/5(vodi)
  [v_q_PCC] -> PC/6(voq)
  Real-Imag to Complex3/1 -> Complex to Magnitude-Angle1/1
  [v_q_PCC] -> Real-Imag to Complex3/2
  [v_d_PCC] -> Real-Imag to Complex3/1
  Zero1/1 -> Assignment/1
  trim_output/1(Out1) -> Terminator/1
  trim_output/2(Out2) -> Terminator3/1
  trim_output/3(Out3) -> Terminator4/1
  trim_output/4(Out4) -> Terminator5/1
  v/1 -> Selector6/1, Selector5/1
  Selector6/1 -> [vqout], trim_output/4(vq)
  Selector5/1 -> [vdout], trim_output/3(vd)
  Memory/1 -> Cast To Double/1
  Selector1/1 -> [P_s_to_follow]
  NOT1/1 -> AND2/1
  [connected] -> NOT1/1
  AND2/1 -> Product1/1, Product2/1
  [connect] -> Scope/1, AND1/1
  [safe_to_connect] -> AND1/2
  AND1/1 -> Integrator/2, Cast To Double2/1
  Cast To Double2/1 -> Integrator/1
  Memory1/1 -> Cast To Boolean/1
  VCC/1(vidref) -> [vod], Reference frame transform3/1(in_d)
  VCC/2(viqref) -> [voq], Reference frame transform3/3(in_q)
  Sum12/1 -> Switch2/3
  Sum1/1 -> Switch2/1, Sum12/2
  [omega_to_follow] -> Sum11/2, Switch3/1
  [connected] -> Switch2/2, Switch3/2
  Sum11/1 -> Switch3/3
  [P_s_to_follow] -> PC/7(Psp)
  [Q_s_to_follow] -> PC/8(Qsp)
  [v_to_follow] -> Sum1/1
  iV/1 -> Sum1/2
  [connect] -> AND2/2
  Switch3/1 -> LPF_omega/1(in)
  Switch2/1 -> LPF_v/1(in)
  PI_synchro_f/1(Out1) -> Sum11/1
  PI_synchro_v/1(Out1) -> Sum12/1
  LPF_v/1(out) -> PC/4(Eref)
  LPF_omega/1(out) -> PC/3(omegaref)
  Selector7/1 -> Sum2/1
  [omega_base] -> Selector8/1
  Product3/1 -> frame/1
  Selector8/1 -> Product3/2
  Sum2/1 -> Product3/1
  PC/4(Q_f) -> [Q_s], [Q_f]
  [omega] -> Matrix Concatenate/1  "omega"
  Integrator/1 -> Compare To Constant3/1
  Compare To Constant3/1 -> connect/3(connect)
  Compare To Constant2/1 -> OR/2
  frame/1 -> Sum/1
  Sum/1 -> [theta]
  PC/3(P_f) -> LPF_P/1(P), [P_s], [P_f]
  Sum4/1 -> Gain/1
  Constant1/1 -> Sum4/2
  LPF_P/1(P_f) -> Sum4/1
  Gain/1 -> Sum/2

== system VFlexP_small/Grid/Dynamic/Generators/IG ==
  note: do not rename this block, conditions to initialise the generator from PF result are set on this block's output
  note: port number 1
  note: port number 2
  elec_in : Inport
  v : Inport  Port=2
  Assignment : Assignment  NumberOfDimensions=2  DiagnosticForDimensions=Warning  IndexOptions=Assign all,Index vector (dialog)  Indices=1,block_idx  OutputSizes=1,1
  Cast To Double : DataTypeConversion  OutDataTypeStr=boolean  SaturateOnIntegerOverflow=off  RndMeth=Floor
  Constant : Constant  Value=zeros(1, length(block_buses))  VectorParams1D=off
  Constant1 : Constant  Value=ones(1, length(block_buses))  VectorParams1D=off
  Display : Display
  For Each Subsystem : Subsystem  TreatAsAtomicUnit=on
  Integrator1 : Integrator  InitialCondition=Grid_op_IG.op.States(1).x'
  Integrator2 : Integrator  InitialCondition=Grid_op_IG.op.States(2).x'
  Matrix Concatenate : Concatenate  NumInputs=6  Mode=Multidimensional array
  Matrix Concatenate1 : Concatenate  NumInputs=3  Mode=Multidimensional array
  Memory2 : Memory  InitialCondition=1
  One : Constant  OutDataTypeStr=Inherit: Inherit via back propagation
  PQ : Subsystem
  Product3 : Product
  RL out : Subsystem  Variant=on  VariantControlMode=label  LabelModeActiveChoice=dynamic  mask{dynamic=Dynamic, R=1e-6, L=1e-6}
      mask prompts: dynamic "Dynamic behavior"; R "Series resistance (p.u.)"; L "Inductance (p.u.)"
      mask init: same as VFlexP_small/Grid/Dynamic/Generators/GFr/RL out
      mask TypeOptions dynamic: Static | Dynamic | Static omega
  Reference frame transform2 : Subsystem
  Selector1 : Selector  InputPortWidth=length(fref.ref_units)  IndexOptions=Index vector (dialog)  Indices=block_fref  OutputSizes=1
  Selector2 : Selector  NumberOfDimensions=2  InputPortWidth=3  IndexOptions=Index vector (dialog),Index vector (dialog)  Indices=3,block_idx  OutputSizes=1,1
  Selector4 : Selector  NumberOfDimensions=2  InputPortWidth=3  IndexOptions=Index vector (dialog),Index vector (dialog)  Indices=5,block_idx  OutputSizes=1,1
  Selector5 : Selector  NumberOfDimensions=2  InputPortWidth=3  IndexOptions=Index vector (dialog),Index vector (dialog)  Indices=1,block_buses  OutputSizes=1,1
  Selector6 : Selector  NumberOfDimensions=2  InputPortWidth=3  IndexOptions=Index vector (dialog),Index vector (dialog)  Indices=2,block_buses  OutputSizes=1,1
  Selector7 : Selector  NumberOfDimensions=2  InputPortWidth=3  IndexOptions=Index vector (dialog),Index vector (dialog)  Indices=6,block_idx  OutputSizes=1,1
  Selector8 : Selector  InputPortWidth=length(fref.ref_units)  IndexOptions=Index vector (dialog)  Indices=block_fref  OutputSizes=1
  Signal Specification : SignalSpecification  Dimensions=[6 length(buses_lf)]
  Signal Specification1 : SignalSpecification  Dimensions=[3 length(block_buses)]
  Sum1 : Sum  Inputs=|-+
  Terminator{,1..6} (7 alike) : Terminator
  Zero1 : Constant  Value=zeros(6, length(buses_lf))  VectorParams1D=off  OutDataTypeStr=Inherit: Inherit via back propagation
  connect : Subsystem
  theta : Integrator  InitialCondition=Grid_op_IG.op.States(7).x'  UpperSaturationLimit=2*pi  LowerSaturationLimit=0
  trim_output : Subsystem
  elec_out : Outport
  i : Outport  Port=2
  wires:
  [vqout] -> RL out/4(v_out_q)
  RL out/3(v_outd) -> Terminator/1
  RL out/4(v_outq) -> Terminator1/1
  Reference frame transform2/1(out_d) -> RL out/1(v_in_d)
  Reference frame transform2/2(out_q) -> RL out/3(v_in_q)
  theta/1 -> Reference frame transform2/2(theta)
  Integrator1/1 -> Reference frame transform2/1(in_d)
  Integrator2/1 -> Reference frame transform2/3(in_q)
  Product3/1 -> theta/1
  Sum1/1 -> Product3/1
  [omega_ref] -> Selector1/1  "ref_omega"
  One/1 -> Sum1/1
  [vdout] -> RL out/2(v_out_d)
  RL out/1(id) -> PQ/2(id), connect/1(id), trim_output/1(id)
  RL out/2(iq) -> PQ/4(iq), connect/2(iq), trim_output/2(iq)
  Matrix Concatenate1/1 -> Signal Specification1/1
  Signal Specification1/1 -> For Each Subsystem/1(In1)
  Constant/1 -> Matrix Concatenate1/3
  For Each Subsystem/1(Out1) -> i/1
  trim_output/3(Out3) -> Terminator4/1
  trim_output/1(Out1) -> Terminator2/1
  trim_output/4(Out4) -> Terminator5/1
  trim_output/2(Out2) -> Terminator3/1
  v/1 -> Selector6/1, Selector5/1
  Selector5/1 -> [vdout], trim_output/3(vd)
  Selector6/1 -> [vqout], trim_output/4(vq)
  elec_in/1 -> Selector7/1, Selector4/1, Selector2/1
  Matrix Concatenate/1 -> Assignment/2
  Zero1/1 -> Assignment/1
  Assignment/1 -> Signal Specification/1
  Constant1/1 -> Matrix Concatenate/1
  Selector2/1 -> Matrix Concatenate/3
  Selector4/1 -> Memory2/1, Matrix Concatenate/5
  Selector7/1 -> Matrix Concatenate/6
  Signal Specification/1 -> Display/1, elec_out/1
  [vdout] -> PQ/1(vd)
  [vqout] -> PQ/3(vq)
  PQ/1(P) -> Matrix Concatenate/2
  PQ/2(Q) -> Matrix Concatenate/4
  [omega_base] -> Selector8/1
  Selector8/1 -> Product3/2
  Selector1/1 -> Sum1/2
  Memory2/1 -> Cast To Double/1
  [connect] -> connect/3(connect)
  connect/2(iq_real) -> Matrix Concatenate1/2
  connect/1(id_real) -> Matrix Concatenate1/1
  connect/3(connected) -> Terminator6/1
  Cast To Double/1 -> [connect]
